simulink model "subsystem_degreeChange"  (R2021a)
settings: Solver=VariableStepAuto  StartTime=0.0  StopTime=10.0  RelTol=1e-3
settings Model: Creator=Beshary  LastModifiedBy=Beshary

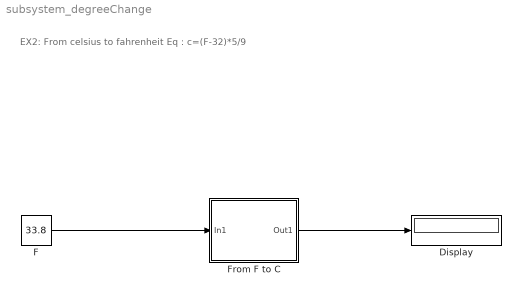
== system subsystem_degreeChange ==
  note: EX2: From celsius to fahrenheit
      | Eq : c=(F-32)*5/9
  Display : Display
  F : Constant  Value=33.8
  From F to C : Subsystem
  wires:
  F/1 -> From F to C/1(In1)
  From F to C/1(Out1) -> Display/1

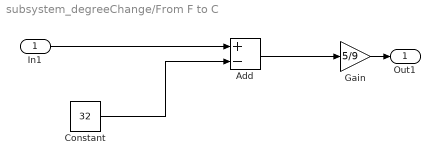
== system subsystem_degreeChange/From F to C ==
  In1 : Inport
  Add : Sum  Inputs=+-
  Constant : Constant  Value=32
  Gain : Gain  Gain=5/9
  Out1 : Outport
  wires:
  Constant/1 -> Add/2
  In1/1 -> Add/1
  Add/1 -> Gain/1
  Gain/1 -> Out1/1
